simulink model "translation"  (R2015a)
settings: Solver=ode45  StartTime=0.0  StopTime=10.0  RelTol=1e-3
undefined symbols (not defined in the file): L1, L12, v
libraries: simulink x2
settings Model: Creator=Sara  LastModifiedBy=Sara

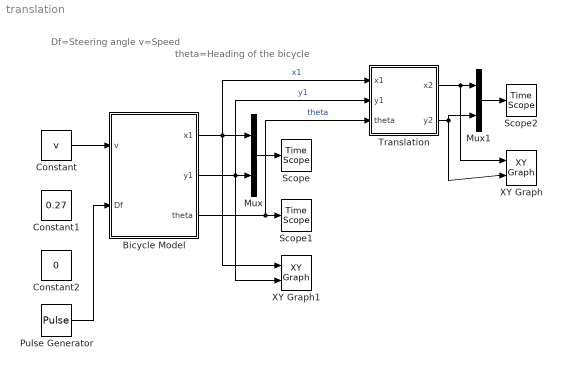
== system translation ==
  note: theta=Heading of the bicycle
  note: Df=Steering angle
      | v=Speed
  Bicycle Model : Subsystem
  Constant : Constant  Value=v
  Constant1 : Constant  Value=0.27
  Constant2 : Constant  Value=0
  Mux : Mux  Inputs=2
  Mux1 : Mux  Inputs=2
  Pulse Generator : DiscretePulseGenerator  PulseType=Time based  Amplitude=0.3  Period=10  PulseWidth=50  PhaseDelay=2
  Scope : TimeScope
  Scope1 : TimeScope
  Scope2 : TimeScope
  Translation : Subsystem
  XY Graph : simulink/Sinks/XY Graph  xmin=-40  xmax=40  ymin=-40  ymax=40  st=-1
  XY Graph1 : simulink/Sinks/XY Graph  xmin=-40  xmax=40  ymin=-40  ymax=40  st=-1
  wires:
  Constant/1 -> Bicycle Model/1(v)
  Bicycle Model/1(x1) -> XY Graph1/1, Translation/1(x1), Mux/1  "x1"
  Bicycle Model/2(y1) -> XY Graph1/2, Translation/2(y1), Mux/2  "y1"
  Mux/1 -> Scope/1
  Bicycle Model/3(theta) -> Translation/3(theta), Scope1/1  "theta"
  Translation/2(y2) -> XY Graph/2, Mux1/2
  Mux1/1 -> Scope2/1
  Translation/1(x2) -> XY Graph/1, Mux1/1
  Pulse Generator/1 -> Bicycle Model/2(Df)

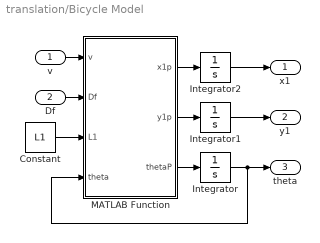
== system translation/Bicycle Model ==
  v : Inport
  Df : Inport  Port=2
  Constant : Constant  Value=L1
  Integrator : Integrator
  Integrator1 : Integrator
  Integrator2 : Integrator
  MATLAB Function : MATLAB Function  TreatAsAtomicUnit=on
  x1 : Outport
  y1 : Outport  Port=2
  theta : Outport  Port=3
  wires:
  MATLAB Function/1(x1p) -> Integrator2/1
  MATLAB Function/3(thetaP) -> Integrator/1
  Integrator1/1 -> y1/1
  v/1 -> MATLAB Function/1(v)
  Integrator2/1 -> x1/1
  Df/1 -> MATLAB Function/2(Df)
  Integrator/1 -> MATLAB Function/4(theta), theta/1
  MATLAB Function/2(y1p) -> Integrator1/1
  Constant/1 -> MATLAB Function/3(L1)

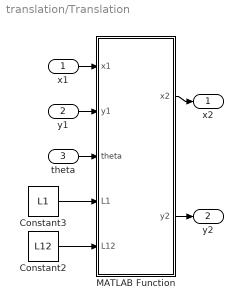
== system translation/Translation ==
  x1 : Inport
  y1 : Inport  Port=2
  theta : Inport  Port=3
  Constant2 : Constant  Value=L12
  Constant3 : Constant  Value=L1
  MATLAB Function : MATLAB Function  TreatAsAtomicUnit=on
  x2 : Outport
  y2 : Outport  Port=2
  wires:
  Constant2/1 -> MATLAB Function/5(L12)
  Constant3/1 -> MATLAB Function/4(L1)
  y1/1 -> MATLAB Function/2(y1)
  x1/1 -> MATLAB Function/1(x1)
  MATLAB Function/1(x2) -> x2/1
  theta/1 -> MATLAB Function/3(theta)
  MATLAB Function/2(y2) -> y2/1

== matlab function translation/Translation/MATLAB Function ==
  data: x1 input; x2 output; y1 input; theta input; L1 input; L12 input; y2 output
function [x2,y2] = fcn(x1,y1,theta,L1,L12)
x2 = x1-(L1+L12)*cos(theta);
y2 = y1-(L1+L12)*sin(theta);

== matlab function translation/Bicycle Model/MATLAB Function ==
  data: x1p output; y1p output; v input; thetaP output; Df input; L1 input; theta input
function [x1p,y1p,thetaP] = fcn(v,Df,L1,theta)
%Rotation rate equation
thetaP=(v*sin(Df))/L1;

x1p=v*cos(theta+Df);
y1p=v*sin(theta+Df);
